simulink model "DCM_measurementMdl"  (R2021a)
settings: Solver=ode1  StartTime=0.0  StopTime=40  FixedStep=Ts  RelTol=1e-3
undefined symbols (not defined in the file or in its folder): National_Instruments, PCIe
libraries: sldrtlib x2, simulink x1
Description:
  | Water Tank Model with Dashboard
  | 
  | The example model "sldrtex_dashboard" shows a real-time model of a water tank
  | controlled by dashboard controls.  You can change the inputs to the plant using
  | the knobs and observe the response on the gauges.
  | 
  | How to run this model in Normal Mode:
  | 
  | 1) Double-click the orange button to switch to Normal Mode if needed.
  | 2) Start the real-time execution using Simulation->Run.
  | 3) Change the input flow and output valve values by the dashboard controls and observe
  |    the results on the dashboard gauges.
  | 
  | How to run this model in External Mode:
  | 
  | 1) Double-click the orange button to switch to External Mode if needed.
  | 2) Start the real-time execution using Simulation->Run. The model will automatically
  |    build, connect to Simulink in External Mode and start.
  | 3) Change the input flow and output valve values by the dashboard controls and observe
  |    the results on the dashboard gauges.
settings Model: SimulationMode=external  ExtModeTrigDuration=100001  Creator=The MathWorks, Inc.  LastModifiedBy=k61432
settings SolverCC: AlgebraicLoopSolver=TrustRegion  AutoInsertRateTranBlk=on
settings DataIOCC: LimitDataPoints=on  SaveFormat=Array  ReturnWorkspaceOutputs=off  SignalLoggingName=logsOut
settings OptimizationCC: ExpressionDepthLimit=2147483647  InitFltsAndDblsToZero=on  EfficientMapNaN2IntZero=off  LifeSpan=inf
settings DebuggingCC: UnderspecifiedInitializationDetection=Classic  MergeDetectMultiDrivingBlocksExec=none  SignalResolutionControl=TryResolveAllWithWarning  FcnCallInpInsideContextMsg=warning  AllowSymbolicDim=off  StateNameClashWarn=warning  SFUnexpectedBacktrackingDiag=warning  SFNoUnconditionalDefaultTransitionDiag=warning  SFExecutionAtInitializationDiag=none  SFMachineParentedDataDiag=warning  ArithmeticOperatorsInVariantConditions=warning
settings HardwareCC: TargetBitPerLong=64  TargetBitPerPointer=64  TargetBitPerSizeT=64  TargetBitPerPtrDiffT=64  TargetIntDivRoundTo=Zero  TargetEndianess=LittleEndian  TargetWordSize=64  TargetHWDeviceType=Intel->x86-64
settings ModelReferenceCC: PropagateSignalLabelsOutOfModel=off
settings SFSimCC: SimUseLocalCustomCode=off  CustomCodeUndefinedFunction=UseInterfaceOnly
settings RTWCC: Description=Simulink Desktop Real-Time  SystemTargetFile=sldrt.tlc  TemplateMakefile=sldrt.tmf  RTWUseLocalCustomCode=off  RTWCompilerOptimization=on
settings CodeAppCC: MaxIdLength=95  StateflowObjectComments=on
settings SimulinkDesktopRealTimeCC: TargetPreCompLibLocation=C:\Program Files\MATLAB\R2021a\toolbox\sldrt\lib\win64  TargetLangStandard=C89/C90 (ANSI)  SupportVariableSizeSignals=off
settings ConfigComp: CovMetricSettings=dw  CovSaveCumulativeToWorkspaceVar=on  CovSaveSingleToWorkspaceVar=on  CovExternalEMLEnable=off  CovSFcnEnable=off

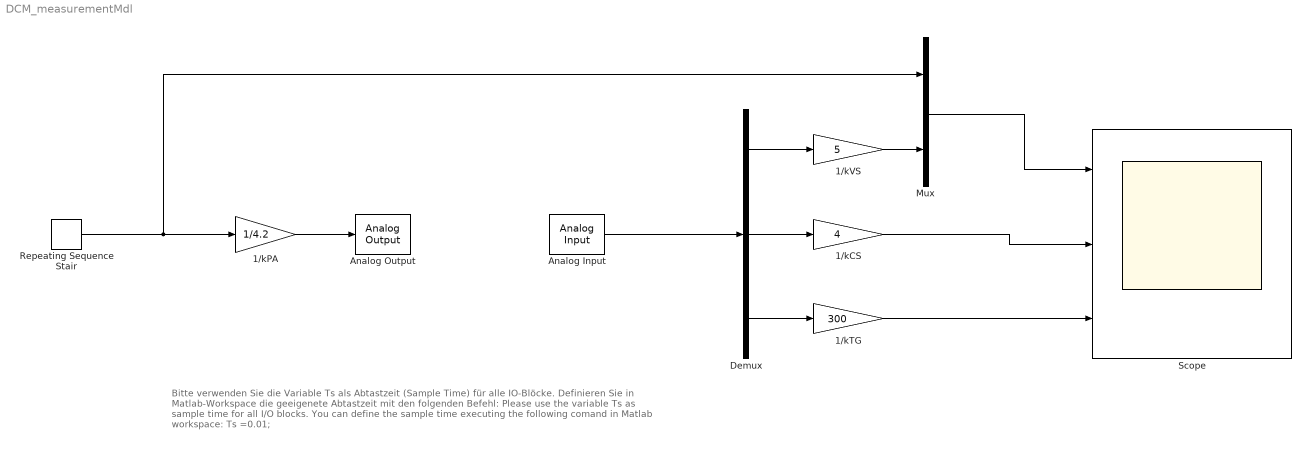
== system DCM_measurementMdl ==
  note: Bitte verwenden Sie die Variable Ts als Abtastzeit (Sample Time) für alle IO-Blöcke. Definieren Sie in Matlab-Workspace die geeigenete Abtastzeit mit den folgenden Befehl:
      | Please use the variable Ts as sample time for all I/O blocks. You can define the sample time executing the following comand in Matlab workspace:
      |   Ts =0.01;
  1/kCS : Gain  Gain=4
  1/kPA : Gain  Gain=1/4.2
  1/kTG : Gain  Gain=300
  1/kVS : Gain  Gain=5
  Analog Input : sldrtlib/Analog Input  SampleTime=0.001  MaxMissedTicks=10  ShowMissedTicks=off  YieldWhenWaiting=off  DrvName=National_Instruments/PCIe-6321  DrvAddress=4294967295  DrvOptions=[0 0 0 0 0 0 0]  Channels=[1 2 3]  RangeMode=1  VoltRange=1  DataType=1
      settings: AttributesFormatString=National Instruments\nPCIe-6321 [auto]
  Analog Output : sldrtlib/Analog Output  SampleTime=0.001  MaxMissedTicks=10  ShowMissedTicks=off  YieldWhenWaiting=off  DrvName=National_Instruments/PCIe-6321  DrvAddress=4294967295  DrvOptions=[0 0 0 0 0 0 0]  Channels=1  RangeMode=1  VoltRange=1  InitialValue=0  FinalValue=0
      settings: AttributesFormatString=National Instruments\nPCIe-6321 [auto]
  Demux : Demux  Outputs=3
  Mux : Mux  Inputs=2
  Repeating Sequence Stair : simulink/Sources/Repeating Sequence Stair  OutValues=[0:5:30]  tsamp=3  OutMin=[]  OutMax=[]  OutDataTypeStr=double  OutputDataTypeScalingMode=double  OutDataType=fixdt(0,8)  ConRadixGroup=Best Precision: Vector-wise  OutScaling=2^-12
  Scope : Scope  NumInputPorts=3
  wires:
  Demux/1 -> 1/kVS/1
  Demux/2 -> 1/kCS/1
  Demux/3 -> 1/kTG/1
  Repeating Sequence Stair/1 -> 1/kPA/1, Mux/1
  1/kPA/1 -> Analog Output/1
  Analog Input/1 -> Demux/1
  1/kVS/1 -> Mux/2
  Mux/1 -> Scope/1
  1/kCS/1 -> Scope/2
  1/kTG/1 -> Scope/3
